simulink model "Observador_reducido_2015"  (R2021a)
settings: Solver=VariableStepAuto  StartTime=0.0  StopTime=10  RelTol=1e-3
values from neighbouring files (symbols this model uses):
  A = [-2 -1;1 0]    [observador_reducido_ex2.m]
  b = [1; 0]    [observador_reducido_ex2.m]
  c = [0 1]    [observador_reducido_ex2.m]
  F = roots([1 10])    [observador_reducido_ex2.m]
  l = 1    [observador_reducido_ex2.m]
  P = inv([c;T])    [observador_reducido_ex2.m]
  T = sylvester(-F,A,l*c)    [observador_reducido_ex2.m]
settings Model: Creator=Sergio  LastModifiedBy=wilso
settings SolverCC: AlgebraicLoopSolver=TrustRegion
settings DebuggingCC: SFMachineParentedDataDiag=warning

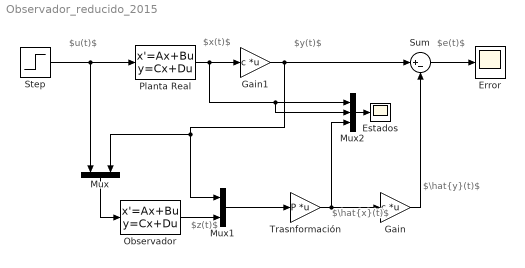
== system Observador_reducido_2015 ==
  note: $\hat{y}(t)$
  note: $y(t)$
  note: $u(t)$
  note: $e(t)$
  note: $\hat{x}(t)$
  note: $x(t)$
  note: $z(t)$
  Error : Scope
  Estados : Scope
  Gain : Gain  Gain=c  Multiplication=Matrix(K*u)
  Gain1 : Gain  Gain=c  Multiplication=Matrix(K*u)
  Mux : Mux  Inputs=2
  Mux1 : Mux  Inputs=2
  Mux2 : Mux  Inputs=3
  Observador : StateSpace  A=F  B=[T*b,l]  D=[0 0]  InitialCondition=0
  Planta Real : StateSpace  A=A  B=b  C=eye(2)  D=[0 0]'  InitialCondition=[-2 1]
  Step : Step  Time=0  SampleTime=0
  Sum : Sum  Inputs=|+-
  Trasnformación : Gain  Gain=P  Multiplication=Matrix(K*u)
  wires:
  Mux/1 -> Observador/1
  Planta Real/1 -> Mux2/2, Mux2/1, Gain1/1
  Step/1 -> Planta Real/1, Mux/1
  Sum/1 -> Error/1
  Gain1/1 -> Mux1/1, Mux/2, Sum/1
  Observador/1 -> Mux1/2
  Mux1/1 -> Trasnformación/1
  Gain/1 -> Sum/2
  Trasnformación/1 -> Mux2/3, Gain/1
  Mux2/1 -> Estados/1
